simulink model "LocalMaxima"  (R2020a)
settings: Solver=VariableStepAuto  StartTime=0.0  StopTime=40  RelTol=1e-3
model workspace (MAT data in the model file):
  a = 0
libraries: simulink x3, dspswit3 x1, dspfdesign x1, hdlsllib x1
settings Model: Creator=sbuccelli  LastModifiedBy=diflo

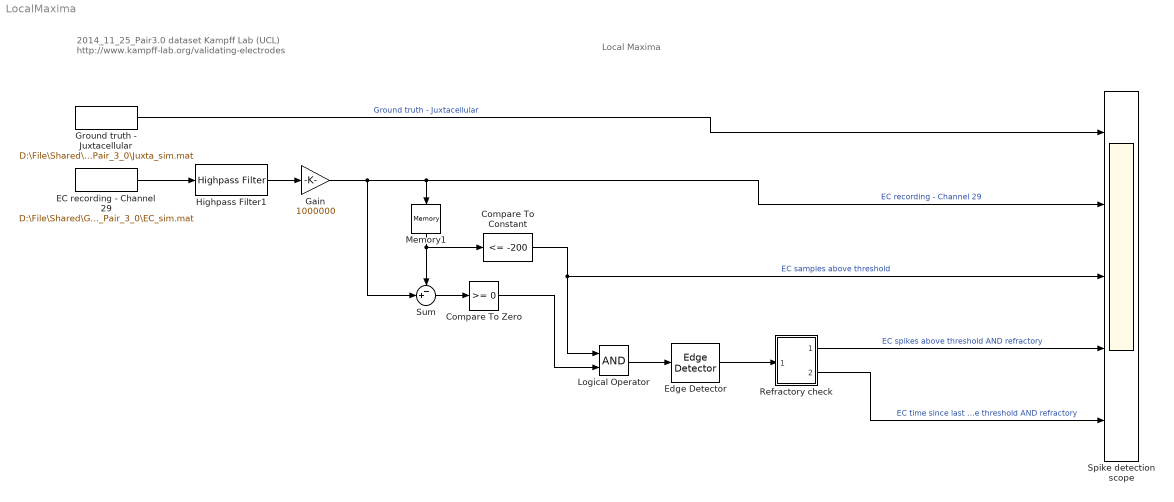
== system LocalMaxima ==
  note: 2014_11_25_Pair3.0 dataset
      | Kampff Lab (UCL)
      | http://www.kampff-lab.org/validating-electrodes
  note: Local Maxima
  Compare To Constant : simulink/Logic and Bit Operations/Compare To Constant  relop=<=  const=-200  OutDataTypeStr=boolean
  Compare To Zero : simulink/Logic and Bit Operations/Compare To Zero  relop=>=  OutDataTypeStr=boolean
  EC recording - Channel 29 : FromFile  FileName=D:\File\Shared\Google Drive\IIT - Neuroengineering\Project\WP1\Data\KampffLab\2014_11_25_Pair_3_0\EC_sim.mat  OutDataTypeStr=double  SampleTime=1/3e4
  Edge Detector : dspswit3/Edge Detector  InputProcessing=Columns as channels (frame based)
      settings: SourceProductBaseCode=DS
  Gain : Gain  Gain=1000000
  Ground truth - Juxtacellular : FromFile  FileName=D:\File\Shared\Google Drive\IIT - Neuroengineering\Project\WP1\Data\KampffLab\2014_11_25_Pair_3_0\Juxta_sim.mat  OutDataTypeStr=double  SampleTime=1/3e4
  Highpass Filter1 : dspfdesign/Highpass Filter  FilterType=IIR  DesignForMinimumOrder=off  FilterOrder=3  StopbandFrequency=1  PassbandFrequency=300  StopbandAttenuation=80  PassbandRipple=0.1  InheritSampleRate=off  SampleRate=30000  SimulateUsing=Interpreted execution  roundingMode=Floor  coeffsDataTypeStr=fixdt(1,16)
  Logical Operator : Logic  AllPortsSameDT=off  OutDataTypeStr=boolean
  Memory1 : Memory  InheritSampleTime=on
  Refractory check : Subsystem
  Spike detection scope : Scope  NumInputPorts=5
  Sum : Sum  Inputs=-+|
  wires:
  EC recording - Channel 29/1 -> Highpass Filter1/1
  Refractory check/1(" ") -> Spike detection scope/4  "EC spikes above threshold AND refractory"
  Refractory check/2(Output) -> Spike detection scope/5  "EC time since last spike above threshold AND refractory"
  Ground truth - Juxtacellular/1 -> Spike detection scope/1  "Ground truth - Juxtacellular"
  Edge Detector/1 -> Refractory check/1("   ")
  Sum/1 -> Compare To Zero/1
  Compare To Constant/1 -> Logical Operator/1, Spike detection scope/3  "EC samples above threshold"
  Logical Operator/1 -> Edge Detector/1
  Compare To Zero/1 -> Logical Operator/2
  Memory1/1 -> Compare To Constant/1, Sum/1
  Highpass Filter1/1 -> Gain/1
  Gain/1 -> Sum/2, Memory1/1, Spike detection scope/2  "EC recording - Channel 29"

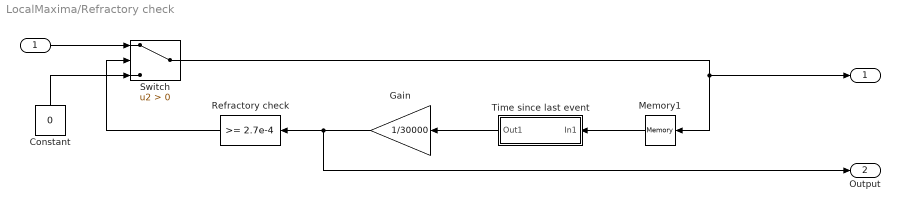
== system LocalMaxima/Refractory check ==
  "   " : Inport
  Constant : Constant  Value=0
  Gain : Gain  Gain=1/30000  ParamDataTypeStr=double
  Memory1 : Memory  InheritSampleTime=on
  Refractory check : simulink/Logic and Bit Operations/Compare To Constant  relop=>=  const=2.7e-4  OutDataTypeStr=boolean
  Switch : Switch  Criteria=u2 > Threshold
  Time since last event : Subsystem
  " " : Outport
  Output : Outport  Port=2
  wires:
  "   "/1 -> Switch/1
  Memory1/1 -> Time since last event/1(In1)
  Time since last event/1(Out1) -> Gain/1
  Constant/1 -> Switch/3
  Gain/1 -> Refractory check/1, Output/1
  Switch/1 -> " "/1, Memory1/1
  Refractory check/1 -> Switch/2

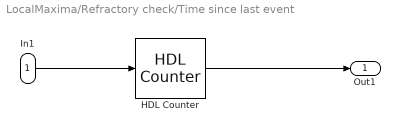
== system LocalMaxima/Refractory check/Time since last event ==
  In1 : Inport
  HDL Counter : hdlsllib/Sources/HDL Counter  CountType=Free running  CountInit=1  CountStep=1  CountMax=25  CountFromType=Initial value  CountFrom=1  CountResetPort=on  CountLoadPort=off  CountEnbPort=off  CountDirPort=off  CountDataType=Unsigned  CountWordLen=32  CountFracLen=0  CountSampTime=1
  Out1 : Outport
  wires:
  In1/1 -> HDL Counter/1
  HDL Counter/1 -> Out1/1
